simulink model "DC_motor_control_loop"  (R2022b)
settings: Solver=ode4  StartTime=0.0  StopTime=100  FixedStep=0.001  MaxStep=0.02  RelTol=1e-3
undefined symbols (not defined in the file or in its folder): myMQTT
libraries: slpidlib x1
settings Model: Creator=Michy  LastModifiedBy=tombach
settings SolverCC: AlgebraicLoopSolver=TrustRegion
settings DataIOCC: ReturnWorkspaceOutputs=off
settings DebuggingCC: UnconnectedInputMsg=warning  UnconnectedOutputMsg=warning  UnconnectedLineMsg=warning  SFMachineParentedDataDiag=warning  ArithmeticOperatorsInVariantConditions=warning
settings HardwareCC: ProdBitPerLong=64  ProdHWDeviceType=Apple->ARM64
settings ModelReferenceCC: EnableRefExpFcnMdlSchedulingChecks=on
settings SFSimCC: SimUseLocalCustomCode=off  CustomCodeUndefinedFunction=UseInterfaceOnly
settings RTWCC: RTWUseLocalCustomCode=off
settings CodeAppCC: StateflowObjectComments=on

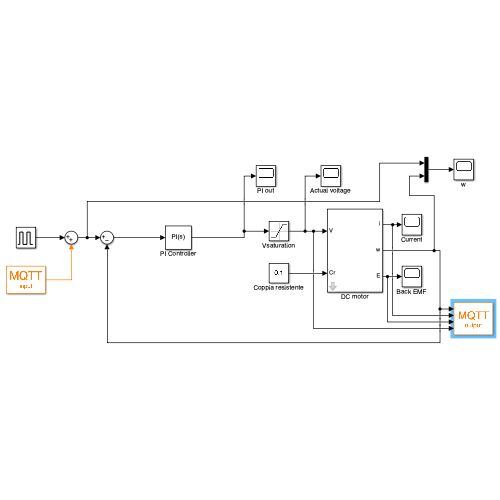
[thumbnail: Simulink's stored preview of the top-level diagram]
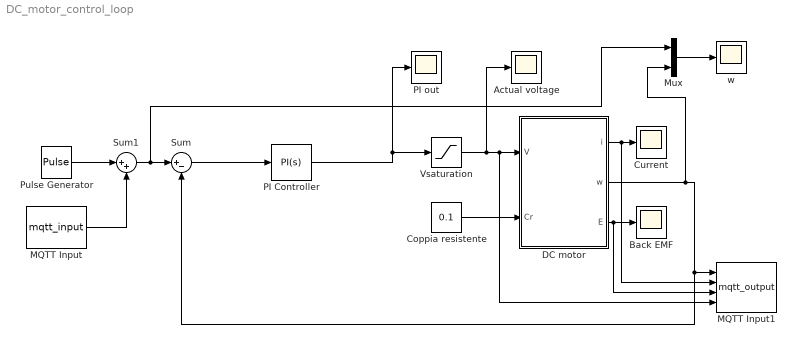
== system DC_motor_control_loop ==
  Actual voltage : Scope
  Back EMF : Scope
  Coppia resistente : Constant  Value=0.1
  Current : Scope
  DC motor : Subsystem  mask{L=0.0028, R=5.5, k=1, phi=0.5, J=0.5}
      mask prompts: L "L [H]"; R "R [Ohm]"; phi "phi [Wb]"; J "J [kg m^2]"
  MQTT Input : M-S-Function  FunctionName=mqtt_input  Parameters=myMQTT,topicName,numOutputs  mask{myMQTT=myMQTT, topicName='test/device1/setpoint', numOutputs=1}
      mask prompts: myMQTT "MQTT Client variable"; topicName "Topic to read messages from"; numOutputs "Number of ouputs"
  MQTT Input1 : M-S-Function  FunctionName=mqtt_output  Parameters=myMQTT,deviceID,topicName,numInputs  mask{myMQTT=myMQTT, deviceID='device1', topicName='test/device1/values', numInputs=4}
      mask prompts: myMQTT "MQTT Client variable"; deviceID "This device ID"; topicName "Topic to write messages to"; numInputs "Number of inputs"
  Mux : Mux  Inputs=2
  PI Controller : slpidlib/PID Controller  Controller=PI  Form=Parallel  TimeDomain=Continuous-time  UseExternalTs=off  SampleTime=-1  IntegratorMethod=Forward Euler  FilterMethod=Forward Euler  ControllerParametersSource=internal  P=5.68484714598179  I=1.72471430989899  UseKiTs=off  D=0  N=100  UseFilter=on  TunerSelectOption=Transfer Function Based (PID Tuner App)  InitialConditionSource=internal  InitialConditionForIntegrator=0  InitialConditionForFilter=0  DifferentiatorICPrevScaledInput=0  ExternalReset=none  TrackingMode=off  Kt=1  LimitOutput=off  SatLimitsSource=internal  UpperSaturationLimit=inf  LowerSaturationLimit=-inf  LinearizeAsGain=on  AntiWindupMode=none  Kb=1  LimitIntegrator=off  UpperIntegratorSaturationLimit=inf  LowerIntegratorSaturationLimit=-inf  POutMin=[]  POutMax=[]  IOutMin=[]  IOutMax=[]  DOutMin=[]  DOutMax=[]  NOutMin=[]  NOutMax=[]  SumOutMin=[]  SumOutMax=[]  SaturationOutMin=[]  SaturationOutMax=[]  PParamMin=[]  PParamMax=[]  IParamMin=[]  IParamMax=[]  DParamMin=[]  DParamMax=[]  NParamMin=[]  NParamMax=[]  KbParamMin=[]  KbParamMax=[]  KtParamMin=[]  KtParamMax=[]  KbOutMin=[]  KbOutMax=[]  KtOutMin=[]  KtOutMax=[]  IntegratorOutMin=[]  IntegratorOutMax=[]  FilterOutMin=[]  FilterOutMax=[]  SumI1OutMin=[]  SumI1OutMax=[]  SumI2OutMin=[]  SumI2OutMax=[]  SumI3OutMin=[]  SumI3OutMax=[]  SumI4OutMin=[]  SumI4OutMax=[]  SumDOutMin=[]  SumDOutMax=[]  DifferentiatorOutMin=[]  DifferentiatorOutMax=[]  FilterDiffOutCoefMin=[]  FilterDiffOutCoefMax=[]  ReciprocalOutMin=[]  ReciprocalOutMax=[]  SumDenOutMin=[]  SumDenOutMax=[]  SumNumOutMin=[]  SumNumOutMax=[]  DivideOutMin=[]  DivideOutMax=[]  UdiffTsProdOutMin=[]  UdiffTsProdOutMax=[]  NTsProdOutMin=[]  NTsProdOutMax=[]  UintegralTsProdOutMin=[]  UintegralTsProdOutMax=[]  UngainTsProdOutMin=[]  UngainTsProdOutMax=[]  ClampingZeroOutDataTypeStr=Inherit: Inherit via back propagation  ClampingZeroOutMin=[]  ClampingZeroOutMax=[]  FilterDenConstantOutDataTypeStr=Inherit: Inherit via back propagation  FilterDenConstantOutMin=[]  FilterDenConstantOutMax=[]  PCopyOutDataTypeStr=Inherit: Inherit via back propagation  PCopyOutMin=[]  PCopyOutMax=[]  NCopyOutDataTypeStr=Inherit: Inherit via back propagation  NCopyOutMin=[]  NCopyOutMax=[]  IntegratorContinuousStateAttributes=''  IntegratorStateMustResolveToSignalObject=off  IntegratorRTWStateStorageClass=Auto  FilterContinuousStateAttributes=''  FilterStateMustResolveToSignalObject=off  FilterRTWStateStorageClass=Auto  ParallelPVariant=InternalParameters  IdealPVariant=Disabled  IVariant=InternalParameters  DVariant=Disabled  IntegratorVariant=Continuous  SatVariant=Disabled  AWVariant=Passthrough  PCopyVariant=Disabled  TRVariant=Disabled  FdbkBlocksVariant=Forward  IdealPFdbkVariant=Disabled  SatFdbkVariant=Disabled  DerivativeFilterVariant=Disabled  NVariant=Disabled  NCopyVariant=Disabled_SignalSpec  FilterICVariant=Disabled  IntegratorICVariant=InternalICs  ExternalResetVariant=Disabled  TRSumVariant=Passthrough  SumFdbkVariant=Disabled  SumVariant=Sum_PI  TsampFilterVariant=InternalTs  TsampNgainVariant=Passthrough  TsampIntegralVariant=Passthrough  ExternalSaturationOutDataTypeStr=Inherit: Same as second input
  PI out : Scope
  Pulse Generator : DiscretePulseGenerator  PulseType=Time based  Amplitude=10  Period=200  PulseWidth=50
  Sum : Sum  Inputs=|+-
  Sum1 : Sum  Inputs=|++
  Vsaturation : Saturate  UpperLimit=24  LowerLimit=0
  w : Scope
  wires:
  Coppia resistente/1 -> DC motor/2(Cr)
  DC motor/2(w) -> Mux/2, Sum/2, MQTT Input1/1
  DC motor/1(i) -> MQTT Input1/2, Current/1
  DC motor/3(E) -> MQTT Input1/3, Back EMF/1
  Vsaturation/1 -> MQTT Input1/4, DC motor/1(V), Actual voltage/1
  PI Controller/1 -> PI out/1, Vsaturation/1
  Sum/1 -> PI Controller/1
  Sum1/1 -> Mux/1, Sum/1
  Mux/1 -> w/1
  MQTT Input/1 -> Sum1/2
  Pulse Generator/1 -> Sum1/1

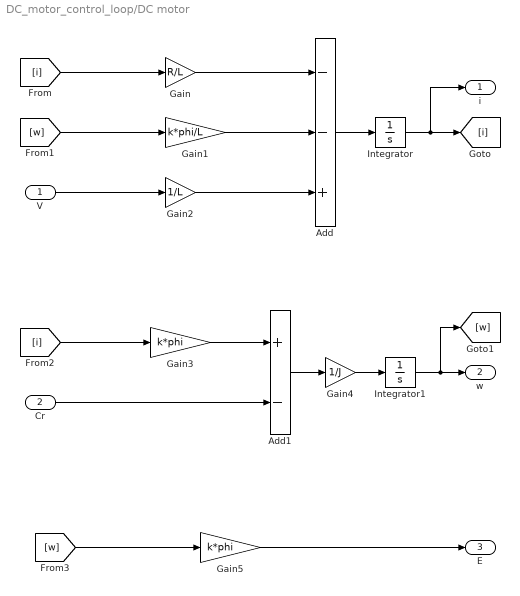
== system DC_motor_control_loop/DC motor ==
  V : Inport
  Cr : Inport  Port=2
  Add : Sum  Inputs=--+
  Add1 : Sum  Inputs=+-
  Gain : Gain  Gain=R/L
  Gain1 : Gain  Gain=k*phi/L
  Gain2 : Gain  Gain=1/L
  Gain3 : Gain  Gain=k*phi
  Gain4 : Gain  Gain=1/J
  Gain5 : Gain  Gain=k*phi
  Integrator : Integrator
  Integrator1 : Integrator
  i : Outport
  w : Outport  Port=2
  E : Outport  Port=3
  wires:
  [i] -> Gain/1
  [w] -> Gain1/1
  V/1 -> Gain2/1
  Gain/1 -> Add/1
  Gain1/1 -> Add/2
  Gain2/1 -> Add/3
  Add/1 -> Integrator/1
  Integrator/1 -> i/1, [i]
  [i] -> Gain3/1
  Gain3/1 -> Add1/1
  Cr/1 -> Add1/2
  Add1/1 -> Gain4/1
  Gain4/1 -> Integrator1/1
  Integrator1/1 -> [w], w/1
  [w] -> Gain5/1
  Gain5/1 -> E/1
